simulink model "transfer"  (R2013a)
settings: Solver=ode45  StartTime=0.0  StopTime=20  RelTol=1e-3
settings Model: Creator=USER  LastModifiedBy=USER

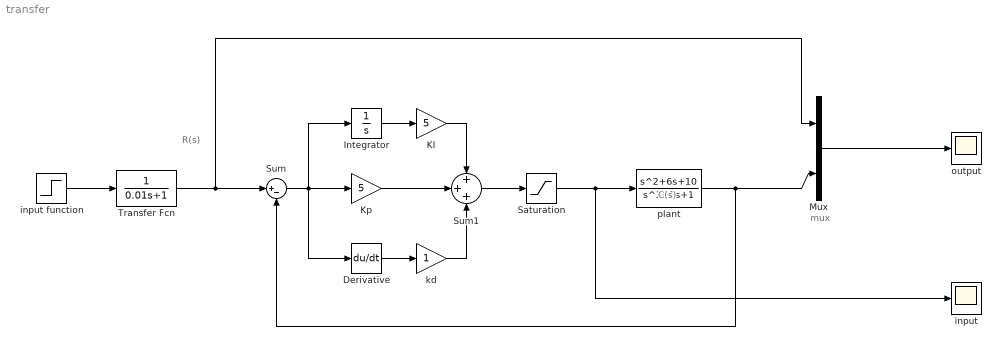
== system transfer ==
  note: C(s)
  note: R(s)
  note: mux
  Derivative : Derivative
  Integrator : Integrator
  "KI " : Gain  Gain=5
  Kp : Gain  Gain=5
  Mux : Mux  Inputs=2
  Saturation : Saturate  UpperLimit=5  LowerLimit=-5
  Sum : Sum  Inputs=|+-
  Sum1 : Sum  Inputs=+++
  Transfer Fcn : TransferFcn  Denominator=[0.01 1]
  input : Scope
      settings: TimeRange=1.237224314147391  YMin=-1.240223463687151  YMax=1.463687150837989
  input function : Step  SampleTime=0
  "kd " : Gain
  "output " : Scope
      settings: TimeRange=1.237224314147391  YMin=-1.240223463687151  YMax=1.463687150837989
  "plant " : TransferFcn  Numerator=[1 6 10]  Denominator=[1 0 7 1]
  wires:
  "plant "/1 -> Mux/2, Sum/2
  input function/1 -> Transfer Fcn/1
  Sum/1 -> Derivative/1, Integrator/1, Kp/1
  Mux/1 -> "output "/1
  Integrator/1 -> "KI "/1
  "KI "/1 -> Sum1/1
  Kp/1 -> Sum1/2
  Sum1/1 -> Saturation/1
  "kd "/1 -> Sum1/3
  Derivative/1 -> "kd "/1
  Transfer Fcn/1 -> Mux/1, Sum/1
  Saturation/1 -> input/1, "plant "/1
